simulink library "dgl_grc"  (R2024a)
settings: Solver=VariableStepAuto  StartTime=0.0  StopTime=10.0  RelTol=1e-3
undefined symbols (not defined in the file or in its folder): Diag2_bRstFault_C, Diag2_f32_UdcLowCoefAddStep_C, Diag2_f32_UdcLowCoefDepStep_C, Diag2_f32_UdcLowHysBand_C, Diag2_f32_UdcLowStartDerat_C, Diag2_f32_UdcLowStopDerat_C, Diag2_f32_UdcOverCoefAddStep_C, Diag2_f32_UdcOverCoefDepStep_C, Diag2_f32_UdcOverHysBand_C, Diag2_f32_UdcOverStartDerat_C, Diag2_f32_UdcOverStopDerat_C, Diag2_int16_HvLowErrErr_C, Diag2_int16_HvLowErrHeal_C, Diag2_int16_HvLowWarnErr_C, Diag2_int16_HvLowWarnHeal_C, Diag2_int16_HvOverErrErr_C, Diag2_int16_HvOverErrHeal_C, Diag2_int16_HvOverWarnErr_C, Diag2_int16_HvOverWarnHeal_C, DiagM_bZeroCurrMor_C, DiagM_bZeroCurrTrig_C, DiagM_Fault2LevelMor_C, DiagM_Fault2LevelTrig_C, GRC_FAKE_SAMPLE_TIME, KDGL_bBusOffEna_C, KDGL_bComInvaildVcuEna_C, KDGL_bComLostVcuEna_C, KDGL_bCurrFaultEna_C, KDGL_bEnaBenchShutDwn_C, KDGL_bEOPFaultEna_C, KDGL_bHvDcVoltFaultEna_C, KDGL_bIGNVoltFaultEna_C, KDGL_bOilTempFaultEna_C, KDGL_bPCBTempFaultEna_C, KDGL_bPosSenrFaultEna_C, KDGL_bPREREGFaultEna_C, KDGL_bRstStallPort_flg, KDGL_bSicFltFaultEna_C, KDGL_bSicTempFaultEna_C, KDGL_bTempSensrFaultEna_C, KDGL_bVCC5VFaultEna_C, KDGL_bVREF5VFaultEna_C, KDGL_bWaterTempFaultEna_C, KDGL_IGBTCoefAddStep_C, KDGL_IGBTCoefDepStep_C, KDGL_IGBTHysBand_C, KDGL_IGBTStartDerat_C, KDGL_IGBTStopDerat_C, KDGL_iMotStallProtEna_A, KDGL_MotCoefAddStep_C, KDGL_MotCoefDepStep_C, KDGL_MotHysBand_C, KDGL_MotStartDerat_C, KDGL_MotStopDerat_C, KDGL_nEOPSpdDiff_rpm, KDGL_nRotStallProtEna_rpm, KDGL_OilCoefAddStep_C, KDGL_OilCoefDepStep_C, KDGL_OilHysBand_C, KDGL_OilStartDerat_C ... (+37)
libraries: Library x28, GRC_Lib x8
(part 1 of 2)
settings Model: Creator=FVT22063  LastModifiedBy=FVT22063

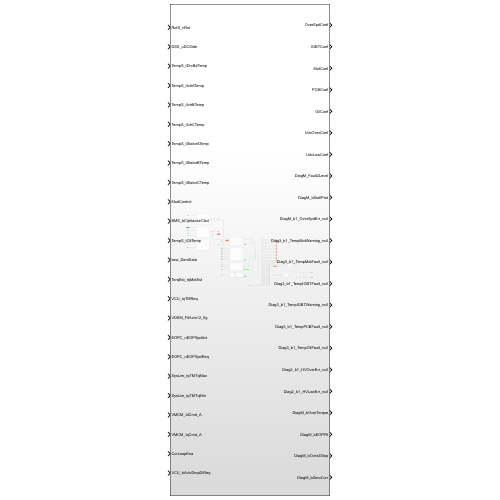
[thumbnail: Simulink's stored preview of the top-level diagram]
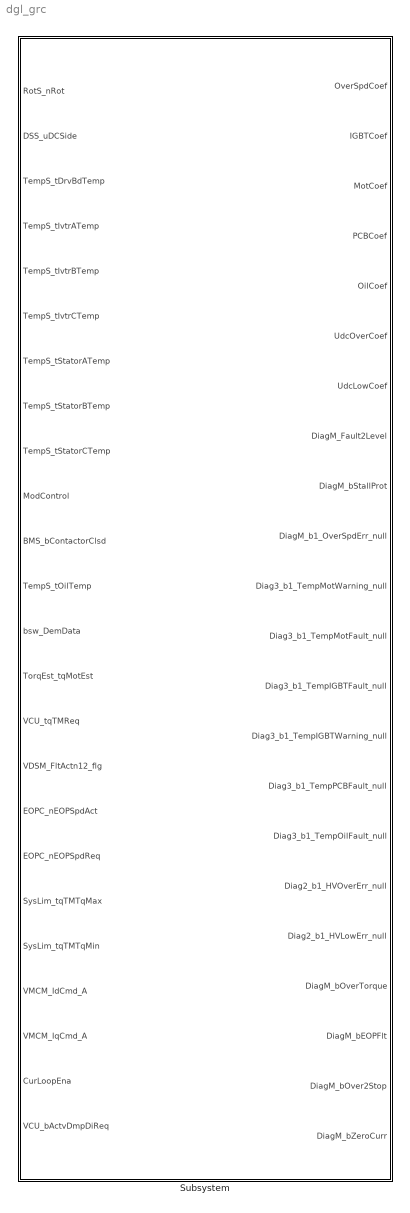
== system dgl_grc ==
  Subsystem : Subsystem

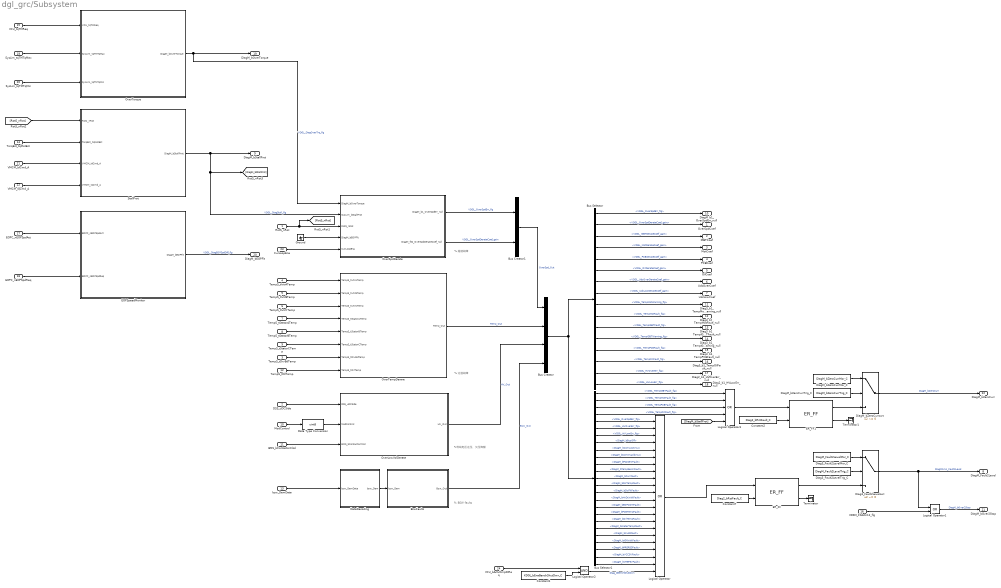
== system dgl_grc/Subsystem ==
  note: % BSW faults
  note: % 超速故障
  note: % 过温故障
  note: %母线电压过压、欠压降额
  RotS_nRot : Inport
  DSS_uDCSide : Inport  Port=2
  TempS_tDrvBdTemp : Inport  Port=3
  TempS_tIvtrATemp : Inport  Port=4
  TempS_tIvtrBTemp : Inport  Port=5
  TempS_tIvtrCTemp : Inport  Port=6
  TempS_tStatorATemp : Inport  Port=7
  TempS_tStatorBTemp : Inport  Port=8
  TempS_tStatorCTemp : Inport  Port=9
  ModControl : Inport  Port=10
  BMS_bContactorClsd : Inport  Port=11
  TempS_tOilTemp : Inport  Port=12
  bsw_DemData : Inport  Port=13  PortDimensions=150
  TorqEst_tqMotEst : Inport  Port=14
  VCU_tqTMReq : Inport  Port=15
  VDSM_FltActn12_flg : Inport  Port=16
  EOPC_nEOPSpdAct : Inport  Port=17
  EOPC_nEOPSpdReq : Inport  Port=18
  SysLim_tqTMTqMax : Inport  Port=19
  SysLim_tqTMTqMin : Inport  Port=20
  VMCM_IdCmd_A : Inport  Port=21
  VMCM_IqCmd_A : Inport  Port=22
  CurLoopEna : Inport  Port=23
  VCU_bActvDmpDiReq : Inport  Port=24
  BswFaults : Subsystem
  Bus Creator : BusCreator  Inputs=4
  Bus Creator1 : BusCreator  Inputs=2
  Bus Selector : BusSelector  OutputSignals=OverSpd_Out.VDGL_OverSpdErr_flg,OverSpd_Out.VDGL_OverSpdDerateCoef_gain,Temp_Out.IGBTTemp.VDGL_IGBTDerateCoef_gain,Temp_Out.StatorTemp.VDGL_MotDerateCoef_gain,Temp_Out.PCBTemp.VDGL_PCBDerateCoef_gain,Temp_Out.OilTemp.VDGL_OilDerateCoef_gain,HV_Out.HVOverMonitor.VDGL_UdcOverDerateCoef_gain,HV_Out.HVLowMonitor.VDGL_UdcLowDerateCoef_gain,Temp_Out.StatorTemp.VDGL_TempMotWarning_flg,Temp_Out.StatorTemp.VDGL_TempMotFault_flg,Temp_Out.IGBTTemp.VDGL_TempIGBTFault_flg,Temp_Out.IGBTTemp.VDGL_TempIGBTWarning_flg,Temp_Out.PCBTemp.VDGL_TempPCBFault_flg,Temp_Out.OilTemp.VDGL_TempOilFault_flg,HV_Out.HVOverMonitor.VDGL_HVOverErr_flg,HV_Out.HVLowMonitor.VDGL_HVLowErr_flg
  Bus Selector1 : BusSelector  OutputSignals=Temp_Out.IGBTTemp.VDGL_TempIGBTFault_flg,Temp_Out.StatorTemp.VDGL_TempMotFault_flg,Temp_Out.PCBTemp.VDGL_TempPCBFault_flg,Temp_Out.OilTemp.VDGL_TempOilFault_flg,OverSpd_Out.VDGL_OverSpdErr_flg,HV_Out.HVOverMonitor.VDGL_HVOverErr_flg,HV_Out.HVLowMonitor.VDGL_HVLowErr_flg,Bsw_Out.DiagM_bBusOff,Bsw_Out.DiagM_bComLostVcu,Bsw_Out.DiagM_bComInvaildVcu,Bsw_Out.DiagM_bPosSenrFault,Bsw_Out.DiagM_bTempSensrFault,Bsw_Out.DiagM_bCurrFault,Bsw_Out.DiagM_bSicTempFault,Bsw_Out.DiagM_bSicFltFault,Bsw_Out.DiagM_bHvDcVoltFault,Bsw_Out.DiagM_bEOPCOMFault,Bsw_Out.DiagM_bPCBTempFault,Bsw_Out.DiagM_bOilTempFault,Bsw_Out.DiagM_bWaterTempFault,Bsw_Out.DiagM_bKL30Fault,Bsw_Out.DiagM_bIGNVoltFault,Bsw_Out.DiagM_bPREREGFault,Bsw_Out.DiagM_bVCC5VFault,Bsw_Out.DiagM_bVREF5VFault
  Constant1 : Constant  Value=KDGL_bEnaBenchShutDwn_C
  Constant2 : Constant  Value=Diag2_bRstFault_C
  Constant7 : Constant  Value=Diag2_bRstFault_C
  Data Type Conversion : DataTypeConversion  OutDataTypeStr=uint8  SaturateOnIntegerOverflow=off  RndMeth=Floor
  DataDecoding : Subsystem
  Diag3_Fault2LevelMor_C : Constant  Value=DiagM_Fault2LevelMor_C
  Diag3_Fault2LevelTrig_C : Constant  Value=DiagM_Fault2LevelTrig_C
  Diag3_Fault2Levelswt : Switch  Criteria=u2 ~= 0  SaturateOnIntegerOverflow=off  InputSameDT=off
  DiagM_bZeroCurrMor_C : Constant  Value=DiagM_bZeroCurrMor_C
  DiagM_bZeroCurrTrig_C : Constant  Value=DiagM_bZeroCurrTrig_C
  DiagM_bZeroCurrswt : Switch  Criteria=u2 ~= 0  SaturateOnIntegerOverflow=off  InputSameDT=off
  EOPSpeedMonitor : Subsystem
  ER_FF : GRC_Lib/Memory/ER_FF  FalseVal=0  TrueVal=1
  ER_FF1 : GRC_Lib/Memory/ER_FF  FalseVal=0  TrueVal=1
  Ground : Ground
  Logical Operator : Logic  Operator=OR  Inputs=22  AllPortsSameDT=off  OutDataTypeStr=boolean
  Logical Operator1 : Logic  Operator=OR  AllPortsSameDT=off  OutDataTypeStr=boolean
  Logical Operator2 : Logic  AllPortsSameDT=off  OutDataTypeStr=boolean
  Logical Operator3 : Logic  Operator=OR  Inputs=5  AllPortsSameDT=off  OutDataTypeStr=boolean
  OverLowVolDerate : Subsystem
  OverSpdDerate : Subsystem
  OverTempDerare : Subsystem
  OverTorque : Subsystem
  StallProt : Subsystem
  Terminator : Terminator
  Terminator1 : Terminator
  OverSpdCoef : Outport  VectorParamsAs1DForOutWhenUnconnected=off
  IGBTCoef : Outport  Port=2  VectorParamsAs1DForOutWhenUnconnected=off
  MotCoef : Outport  Port=3  VectorParamsAs1DForOutWhenUnconnected=off
  PCBCoef : Outport  Port=4  VectorParamsAs1DForOutWhenUnconnected=off
  OilCoef : Outport  Port=5  VectorParamsAs1DForOutWhenUnconnected=off
  UdcOverCoef : Outport  Port=6  VectorParamsAs1DForOutWhenUnconnected=off
  UdcLowCoef : Outport  Port=7  VectorParamsAs1DForOutWhenUnconnected=off
  DiagM_Fault2Level : Outport  Port=8  VectorParamsAs1DForOutWhenUnconnected=off
  DiagM_bStallProt : Outport  Port=9  VectorParamsAs1DForOutWhenUnconnected=off
  DiagM_b1_OverSpdErr_null : Outport  Port=10  VectorParamsAs1DForOutWhenUnconnected=off
  Diag3_b1_TempMotWarning_null : Outport  Port=11  VectorParamsAs1DForOutWhenUnconnected=off
  Diag3_b1_TempMotFault_null : Outport  Port=12  VectorParamsAs1DForOutWhenUnconnected=off
  Diag3_b1_TempIGBTFault_null : Outport  Port=13  VectorParamsAs1DForOutWhenUnconnected=off
  Diag3_b1_TempIGBTWarning_null : Outport  Port=14  VectorParamsAs1DForOutWhenUnconnected=off
  Diag3_b1_TempPCBFault_null : Outport  Port=15  VectorParamsAs1DForOutWhenUnconnected=off
  Diag3_b1_TempOilFault_null : Outport  Port=16  VectorParamsAs1DForOutWhenUnconnected=off
  Diag2_b1_HVOverErr_null : Outport  Port=17  VectorParamsAs1DForOutWhenUnconnected=off
  Diag2_b1_HVLowErr_null : Outport  Port=18  VectorParamsAs1DForOutWhenUnconnected=off
  DiagM_bOverTorque : Outport  Port=19  VectorParamsAs1DForOutWhenUnconnected=off
  DiagM_bEOPFlt : Outport  Port=20  VectorParamsAs1DForOutWhenUnconnected=off
  DiagM_bOver2Stop : Outport  Port=21  VectorParamsAs1DForOutWhenUnconnected=off
  DiagM_bZeroCurr : Outport  Port=22  VectorParamsAs1DForOutWhenUnconnected=off
  wires:
  DiagM_bZeroCurrswt/1 -> DiagM_bZeroCurr/1  "DiagM_bZeroCurr"
  Bus Selector1/6 -> Logical Operator/2  "<VDGL_HVOverErr_flg>"
  [DiagM_bStallProt] -> Logical Operator3/5
  StallProt/1(DiagM_bStallProt) -> [DiagM_bStallProt], OverSpdDerate/2(SysLim_bStallProt), DiagM_bStallProt/1  "VDGL_DiagStall_flg"
  Bus Selector/16 -> Diag2_b1_HVLowErr_null/1  "<VDGL_HVLowErr_flg>"
  Bus Selector1/18 -> Logical Operator/14  "<DiagM_bPCBTempFault>"
  Logical Operator3/1 -> ER_FF1/1
  Bus Selector1/19 -> Logical Operator/15  "<DiagM_bOilTempFault>"
  ER_FF1/1 -> DiagM_bZeroCurrswt/3
  ER_FF1/2 -> Terminator1/1
  ER_FF/1 -> Diag3_Fault2Levelswt/3
  Bus Selector/9 -> Diag3_b1_TempMotWarning_null/1  "<VDGL_TempMotWarning_flg>"
  Diag3_Fault2LevelTrig_C/1 -> Diag3_Fault2Levelswt/2
  TempS_tStatorBTemp/1 -> OverTempDerare/5(TempS_tStatorBTemp)
  Diag3_Fault2LevelMor_C/1 -> Diag3_Fault2Levelswt/1
  VMCM_IdCmd_A/1 -> StallProt/3(VMCM_IdCmd_A)
  Ground/1 -> OverSpdDerate/4(DiagM_bEOPFlt)
  Logical Operator2/1 -> Logical Operator/22  "Diag_bBenchShutDwn"
  Bus Selector/13 -> Diag3_b1_TempPCBFault_null/1  "<VDGL_TempPCBFault_flg>"
  Constant7/1 -> ER_FF/2
  CurLoopEna/1 -> OverSpdDerate/5(CurLoopEna)
  ModControl/1 -> Data Type Conversion/1
  BswFaults/1(Bsw_Out) -> Bus Creator/4  "Bsw_Out"
  Constant1/1 -> Logical Operator2/2
  SysLim_tqTMTqMax/1 -> OverTorque/2(SysLim_tqTMTqMax)
  EOPC_nEOPSpdReq/1 -> EOPSpeedMonitor/2(EOPC_nEOPSpdReq)
  EOPSpeedMonitor/1(DiagM_bEOPFlt) -> DiagM_bEOPFlt/1  "VDGL_DiagEOPSpdDiff_flg"
  SysLim_tqTMTqMin/1 -> OverTorque/3("SysLim_tqTMTqMin ")
  EOPC_nEOPSpdAct/1 -> EOPSpeedMonitor/1(EOPC_nEOPSpdAct)
  Bus Selector/1 -> DiagM_b1_OverSpdErr_null/1  "<VDGL_OverSpdErr_flg>"
  DataDecoding/1(bsw_Dem) -> BswFaults/1(bsw_Dem)
  TorqEst_tqMotEst/1 -> StallProt/2(TorqEst_tqMotEst)
  Diag3_Fault2Levelswt/1 -> Logical Operator1/1, DiagM_Fault2Level/1  "DiagM1ms_Fault2Level"
  Bus Selector1/5 -> Logical Operator/1  "<VDGL_OverSpdErr_flg>"
  Bus Selector/12 -> Diag3_b1_TempIGBTWarning_null/1  "<VDGL_TempIGBTWarning_flg>"
  VCU_bActvDmpDiReq/1 -> Logical Operator2/1
  Logical Operator1/1 -> DiagM_bOver2Stop/1  "DiagM_bOver2Stop"
  Bus Selector1/14 -> Logical Operator/10  "<DiagM_bSicTempFault>"
  VCU_tqTMReq/1 -> OverTorque/1(VCU_tqTMReq)
  OverTorque/1(DiagM_bOverTorque) -> OverSpdDerate/1(DiagM_bOverTorque), DiagM_bOverTorque/1  "VDGL_DiagOverTrq_flg"
  DiagM_bZeroCurrMor_C/1 -> DiagM_bZeroCurrswt/1
  Bus Selector/2 -> OverSpdCoef/1  "<VDGL_OverSpdDerateCoef_gain>"
  Data Type Conversion/1 -> OverLowVolDerate/2(ModControl)
  VDSM_FltActn12_flg/1 -> Logical Operator1/2
  Bus Selector1/24 -> Logical Operator/20  "<DiagM_bVCC5VFault>"
  OverLowVolDerate/1(HV_Out) -> Bus Creator/3  "HV_Out"
  TempS_tIvtrCTemp/1 -> OverTempDerare/3(TempS_tIvtrCTemp)
  bsw_DemData/1 -> DataDecoding/1(bsw_DemData)
  ER_FF/2 -> Terminator/1
  Bus Selector1/21 -> Logical Operator/17  "<DiagM_bKL30Fault>"
  TempS_tOilTemp/1 -> OverTempDerare/8(TempS_tOilTemp)
  VMCM_IqCmd_A/1 -> StallProt/4(VMCM_IqCmd_A)
  RotS_nRot/1 -> [RotS_nRot], OverSpdDerate/3(RotS_nRot)
  Bus Selector1/12 -> Logical Operator/8  "<DiagM_bTempSensrFault>"
  Bus Selector/10 -> Diag3_b1_TempMotFault_null/1  "<VDGL_TempMotFault_flg>"
  Bus Selector1/20 -> Logical Operator/16  "<DiagM_bWaterTempFault>"
  Bus Selector1/10 -> Logical Operator/6  "<DiagM_bComInvaildVcu>"
  OverSpdDerate/2(DiagM_f32_OverSpdDerateCoef_null) -> Bus Creator1/2  "VDGL_OverSpdDerateCoef_gain"
  Bus Selector/14 -> Diag3_b1_TempOilFault_null/1  "<VDGL_TempOilFault_flg>"
  Bus Selector1/7 -> Logical Operator/3  "<VDGL_HVLowErr_flg>"
  Bus Selector1/25 -> Logical Operator/21  "<DiagM_bVREF5VFault>"
  Bus Selector1/23 -> Logical Operator/19  "<DiagM_bPREREGFault>"
  Bus Selector/15 -> Diag2_b1_HVOverErr_null/1  "<VDGL_HVOverErr_flg>"
  Bus Selector1/3 -> Logical Operator3/3  "<VDGL_TempPCBFault_flg>"
  Bus Selector/8 -> UdcLowCoef/1  "<VDGL_UdcLowDerateCoef_gain>"
  Constant2/1 -> ER_FF1/2
  OverTempDerare/1(Temp_Out) -> Bus Creator/2  "Temp_Out"
  [RotS_nRot] -> StallProt/1(Rots_nRot)
  Bus Selector1/4 -> Logical Operator3/4  "<VDGL_TempOilFault_flg>"
  Bus Selector1/17 -> Logical Operator/13  "<DiagM_bEOPCOMFault>"
  OverSpdDerate/1(DiagM_b1_OverSpdErr_null) -> Bus Creator1/1  "VDGL_OverSpdErr_flg"
  Bus Selector/5 -> PCBCoef/1  "<VDGL_PCBDerateCoef_gain>"
  TempS_tIvtrBTemp/1 -> OverTempDerare/2(TempS_tIvtrBTemp)
  BMS_bContactorClsd/1 -> OverLowVolDerate/3(BMS_bContactorClsd)
  Logical Operator/1 -> ER_FF/1
  Bus Selector1/2 -> Logical Operator3/2  "<VDGL_TempMotFault_flg>"
  Bus Selector/7 -> UdcOverCoef/1  "<VDGL_UdcOverDerateCoef_gain>"
  Bus Selector1/15 -> Logical Operator/11  "<DiagM_bSicFltFault>"
  Bus Selector1/11 -> Logical Operator/7  "<DiagM_bPosSenrFault>"
  Bus Selector/6 -> OilCoef/1  "<VDGL_OilDerateCoef_gain>"
  DSS_uDCSide/1 -> OverLowVolDerate/1(DSS_uDCSide)
  Bus Selector1/13 -> Logical Operator/9  "<DiagM_bCurrFault>"
  Bus Selector/4 -> MotCoef/1  "<VDGL_MotDerateCoef_gain>"
  Bus Selector/3 -> IGBTCoef/1  "<VDGL_IGBTDerateCoef_gain>"
  Bus Selector1/9 -> Logical Operator/5  "<DiagM_bComLostVcu>"
  Bus Selector1/16 -> Logical Operator/12  "<DiagM_bHvDcVoltFault>"
  Bus Selector1/8 -> Logical Operator/4  "<DiagM_bBusOff>"
  Bus Creator/1 -> Bus Selector1/1, Bus Selector/1
  Bus Creator1/1 -> Bus Creator/1  "OverSpd_Out"
  TempS_tStatorCTemp/1 -> OverTempDerare/6(TempS_tStatorCTemp)
  Bus Selector1/22 -> Logical Operator/18  "<DiagM_bIGNVoltFault>"
  TempS_tIvtrATemp/1 -> OverTempDerare/1(TempS_tIvtrATemp)
  DiagM_bZeroCurrTrig_C/1 -> DiagM_bZeroCurrswt/2
  TempS_tDrvBdTemp/1 -> OverTempDerare/7(TempS_tDrvBdTemp)
  Bus Selector/11 -> Diag3_b1_TempIGBTFault_null/1  "<VDGL_TempIGBTFault_flg>"
  TempS_tStatorATemp/1 -> OverTempDerare/4(TempS_tStatorATemp)
  Bus Selector1/1 -> Logical Operator3/1  "<VDGL_TempIGBTFault_flg>"

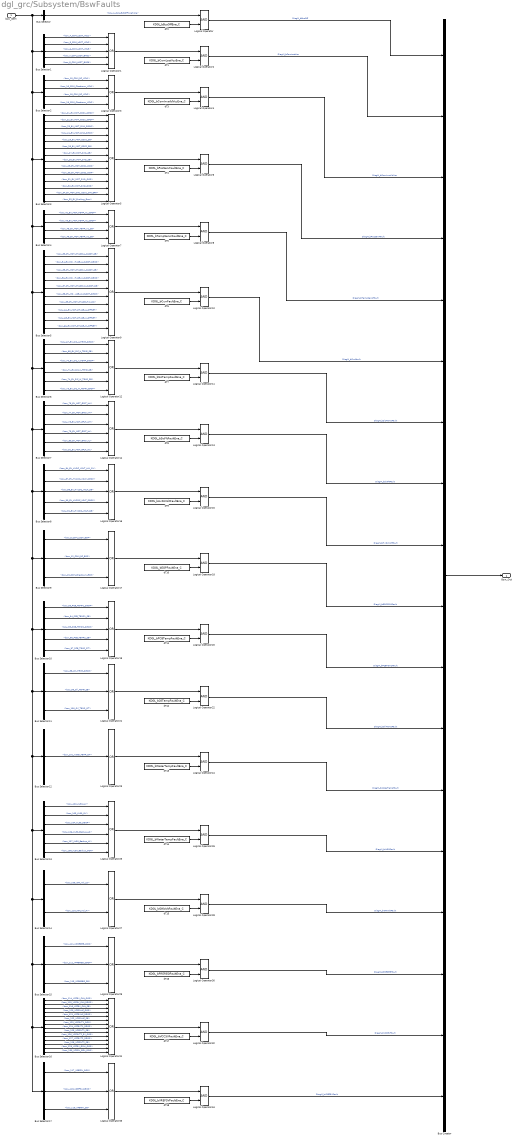
== system dgl_grc/Subsystem/BswFaults ==
  bsw_Dem : Inport
  Bus Creator : BusCreator  Inputs=18
  Bus Selector : BusSelector  OutputSignals=bsw_1_CAN_BUSOFF_Vehicle
  Bus Selector1 : BusSelector  OutputSignals=bsw_4_COM_LOST_VCU1,bsw_5_COM_LOST_VCU2,bsw_6_COM_LOST_VCU5,bsw_7_COM_LOST_BMS1,bsw_8_COM_LOST_BMS6
  Bus Selector10 : BusSelector  OutputSignals=bsw_93_PCB_TEMP1_SGOP,bsw_94_PCB_TEMP1_SB,bsw_95_PCB_TEMP2_SGOP,bsw_96_PCB_TEMP2_SB,bsw_97_PCB_TEMP_OT
  Bus Selector11 : BusSelector  OutputSignals=bsw_98_Oil_TEMP_SGOP,bsw_99_Oil_TEMP_SB,bsw_100_Oil_TEMP_OT
  Bus Selector12 : BusSelector  OutputSignals=bsw_101_water_TEMP_OT
  Bus Selector13 : BusSelector  OutputSignals=bsw_102_KL30_UV,bsw_103_KL30_OV,bsw_104_KL30_SGOP,bsw_106_KL30_Backup_LO,bsw_107_KL30_Backup_HI,bsw_108_KL30_Backup_OOR
  Bus Selector14 : BusSelector  OutputSignals=bsw_109_IGN_Vol_LO,bsw_110_IGN_Vol_HI
  Bus Selector15 : BusSelector  OutputSignals=bsw_111_VPREREG_OOR,bsw_112_VPREREG_SGOP,bsw_113_VPREREG_SB
  Bus Selector16 : BusSelector  OutputSignals=bsw_114_VCC5V_CAN_OOR,bsw_115_VCC5V_CAN_SGOP,bsw_116_VCC5V_CAN_SB,bsw_120_VCC5VUC_OOR,bsw_121_VCC5VUC_SGOP,bsw_122_VCC5VUC_SB,bsw_123_VCC5VT1_OOR,bsw_124_VCC5VT1_SGOP,bsw_125_VCC5VT1_SB,bsw_126_VCC5VT2_5V_OOR,bsw_127_VCC5VT2_SGOP,bsw_128_VCC5VT2_SB,bsw_129_VCC5V_GDH_OOR,bsw_130_VCC5V_GDL_OOR
  Bus Selector17 : BusSelector  OutputSignals=bsw_117_VREF5V_OOR,bsw_118_VREF5V_SGOP,bsw_119_VREF5V_SB
  Bus Selector2 : BusSelector  OutputSignals=bsw_15_COM_RC_VCU1,bsw_16_COM_Checksum_VCU1,bsw_18_COM_RC_VCU2,bsw_19_COM_Checksum_VCU2
  Bus Selector3 : BusSelector  OutputSignals=bsw_21_EV_MOT_COS1_SGOP,bsw_22_EV_MOT_COS2_SGOP,bsw_23_EV_MOT_SIN1_SGOP,bsw_24_EV_MOT_SIN2_SGOP,bsw_25_EV_MOT_COS1_SB,bsw_26_EV_MOT_COS2_SB,bsw_27_EV_MOT_SIN1_SB,bsw_28_EV_MOT_SIN2_SB,bsw_29_EV_MOT_COS1_OOR,bsw_30_EV_MOT_COS2_OOR,bsw_31_EV_MOT_SIN1_OOR,bsw_32_EV_MOT_SIN2_OOR,bsw_34_EV_MOT_SIN1_COS1_DIR_ERR,bsw_33_EV_Exciting_Error
  Bus Selector4 : BusSelector  OutputSignals=bsw_42_EV_MOT_TEMP_V1_SGOP,bsw_43_EV_MOT_TEMP_V2_SGOP,bsw_45_EV_MOT_TEMP_V1_SB,bsw_46_EV_MOT_TEMP_V2_SB
  Bus Selector5 : BusSelector  OutputSignals=bsw_53_EV_MOT_PHASE_U_CURRT_SB,bsw_54_EV_MOT_PHASE_U_CURRT_SGOP,bsw_55_EV_MOT_PHASE_V_CURRT_SB,bsw_56_EV_MOT_PHASE_V_CURRT_SGOP,bsw_57_EV_MOT_PHASE_W_CURRT_SB,bsw_58_EV_MOT_PHASE_W_CURRT_SGOP,bsw_59_EV_MOT_PHASE_HW_OC,bsw_64_EV_MOT_PHASE_U_OFFSET,bsw_65_EV_MOT_PHASE_V_OFFSET,bsw_66_EV_MOT_PHASE_W_OFFSET
  Bus Selector6 : BusSelector  OutputSignals=bsw_67_EV_SIC_U_TEMP_SGOP,bsw_68_EV_SIC_U_TEMP_SB,bsw_70_EV_SIC_V_TEMP_SGOP,bsw_71_EV_SIC_V_TEMP_SB,bsw_74_EV_SIC_W_TEMP_SB,bsw_73_EV_SIC_W_TEMP_SGOP
  Bus Selector7 : BusSelector  OutputSignals=bsw_76_EV_MOT_GFLT_UH,bsw_77_EV_MOT_GFLT_VH,bsw_78_EV_MOT_GFLT_WH,bsw_79_EV_MOT_GFLT_UL,bsw_80_EV_MOT_GFLT_VL,bsw_81_EV_MOT_GFLT_WL
  Bus Selector8 : BusSelector  OutputSignals=bsw_84_EV_HVDC_VOLT_HW_OV,bsw_87_EV_HV1DC_VOLT_SGOP,bsw_88_EV_HV1DC_VOLT_SB,bsw_90_EV_HV2DC_VOLT_SGOP,bsw_91_EV_HV2DC_VOLT_SB
  Bus Selector9 : BusSelector  OutputSignals=bsw_9_COM_LOST_EOP,bsw_12_COM_RC_EOP,bsw_13_COM_Checksum_EOP
  Logical Operator{,2,4,6,8,10..11,13,15,18,20,22,24,26,28,30,32,34} (18 alike) : Logic  AllPortsSameDT=off  OutDataTypeStr=boolean
  Logical Operator1 : Logic  Operator=OR  Inputs=5  AllPortsSameDT=off  OutDataTypeStr=boolean
  Logical Operator12 : Logic  Operator=OR  Inputs=6  AllPortsSameDT=off  OutDataTypeStr=boolean
  Logical Operator14 : Logic  Operator=OR  Inputs=6  AllPortsSameDT=off  OutDataTypeStr=boolean
  Logical Operator16 : Logic  Operator=OR  Inputs=5  AllPortsSameDT=off  OutDataTypeStr=boolean
  Logical Operator{17,21,29,33} (4 alike) : Logic  Operator=OR  Inputs=3  AllPortsSameDT=off  OutDataTypeStr=boolean
  Logical Operator19 : Logic  Operator=OR  Inputs=5  AllPortsSameDT=off  OutDataTypeStr=boolean
  Logical Operator23 : Logic  Operator=OR  Inputs=1  AllPortsSameDT=off  OutDataTypeStr=boolean
  Logical Operator25 : Logic  Operator=OR  Inputs=6  AllPortsSameDT=off  OutDataTypeStr=boolean
  Logical Operator27 : Logic  Operator=OR  AllPortsSameDT=off  OutDataTypeStr=boolean
  Logical Operator3 : Logic  Operator=OR  Inputs=4  AllPortsSameDT=off  OutDataTypeStr=boolean
  Logical Operator31 : Logic  Operator=OR  Inputs=14  AllPortsSameDT=off  OutDataTypeStr=boolean
  Logical Operator5 : Logic  Operator=OR  Inputs=14  AllPortsSameDT=off  OutDataTypeStr=boolean
  Logical Operator7 : Logic  Operator=OR  Inputs=4  AllPortsSameDT=off  OutDataTypeStr=boolean
  Logical Operator9 : Logic  Operator=OR  Inputs=10  AllPortsSameDT=off  OutDataTypeStr=boolean
  dT1 : Constant  Value=KDGL_bComLostVcuEna_C  OutDataTypeStr=single
  dT10 : Constant  Value=KDGL_bEOPFaultEna_C  OutDataTypeStr=single
  dT11 : Constant  Value=KDGL_bPCBTempFaultEna_C  OutDataTypeStr=single
  dT12 : Constant  Value=KDGL_bOilTempFaultEna_C  OutDataTypeStr=single
  dT13 : Constant  Value=KDGL_bWaterTempFaultEna_C  OutDataTypeStr=single
  dT14 : Constant  Value=KDGL_bWaterTempFaultEna_C  OutDataTypeStr=single
  dT15 : Constant  Value=KDGL_bIGNVoltFaultEna_C  OutDataTypeStr=single
  dT16 : Constant  Value=KDGL_bPREREGFaultEna_C  OutDataTypeStr=single
  dT17 : Constant  Value=KDGL_bVCC5VFaultEna_C  OutDataTypeStr=single
  dT18 : Constant  Value=KDGL_bVREF5VFaultEna_C  OutDataTypeStr=single
  dT2 : Constant  Value=KDGL_bBusOffEna_C  OutDataTypeStr=single
  dT3 : Constant  Value=KDGL_bComInvaildVcuEna_C  OutDataTypeStr=single
  dT4 : Constant  Value=KDGL_bPosSenrFaultEna_C  OutDataTypeStr=single
  dT5 : Constant  Value=KDGL_bTempSensrFaultEna_C  OutDataTypeStr=single
  dT6 : Constant  Value=KDGL_bCurrFaultEna_C  OutDataTypeStr=single
  dT7 : Constant  Value=KDGL_bSicTempFaultEna_C  OutDataTypeStr=single
  dT8 : Constant  Value=KDGL_bSicFltFaultEna_C  OutDataTypeStr=single
  dT9 : Constant  Value=KDGL_bHvDcVoltFaultEna_C  OutDataTypeStr=single
  Bsw_Out : Outport  VectorParamsAs1DForOutWhenUnconnected=off
  wires:
  Bus Creator/1 -> Bsw_Out/1
  Bus Selector/1 -> Logical Operator/1  "<bsw_1_CAN_BUSOFF_Vehicle>"
  Logical Operator/1 -> Bus Creator/1  "DiagM_bBusOff"
  dT2/1 -> Logical Operator/2
  Bus Selector1/1 -> Logical Operator1/1  "<bsw_4_COM_LOST_VCU1>"
  Bus Selector1/2 -> Logical Operator1/2  "<bsw_5_COM_LOST_VCU2>"
  Bus Selector1/3 -> Logical Operator1/3  "<bsw_6_COM_LOST_VCU5>"
  Bus Selector1/4 -> Logical Operator1/4  "<bsw_7_COM_LOST_BMS1>"
  Bus Selector1/5 -> Logical Operator1/5  "<bsw_8_COM_LOST_BMS6>"
  dT1/1 -> Logical Operator2/2
  Logical Operator1/1 -> Logical Operator2/1
  Logical Operator2/1 -> Bus Creator/2  "DiagM_bComLostVcu"
  Bus Selector2/3 -> Logical Operator3/3  "<bsw_18_COM_RC_VCU2>"
  Bus Selector2/2 -> Logical Operator3/2  "<bsw_16_COM_Checksum_VCU1>"
  Bus Selector2/4 -> Logical Operator3/4  "<bsw_19_COM_Checksum_VCU2>"
  Bus Selector2/1 -> Logical Operator3/1  "<bsw_15_COM_RC_VCU1>"
  dT3/1 -> Logical Operator4/2
  Logical Operator3/1 -> Logical Operator4/1
  Logical Operator4/1 -> Bus Creator/3  "DiagM_bComInvaildVcu"
  Bus Selector3/1 -> Logical Operator5/1  "<bsw_21_EV_MOT_COS1_SGOP>"
  Bus Selector3/2 -> Logical Operator5/2  "<bsw_22_EV_MOT_COS2_SGOP>"
  Bus Selector3/3 -> Logical Operator5/3  "<bsw_23_EV_MOT_SIN1_SGOP>"
  Bus Selector3/4 -> Logical Operator5/4  "<bsw_24_EV_MOT_SIN2_SGOP>"
  Bus Selector3/5 -> Logical Operator5/5  "<bsw_25_EV_MOT_COS1_SB>"
  Bus Selector3/6 -> Logical Operator5/6  "<bsw_26_EV_MOT_COS2_SB>"
  Bus Selector3/7 -> Logical Operator5/7  "<bsw_27_EV_MOT_SIN1_SB>"
  Bus Selector3/8 -> Logical Operator5/8  "<bsw_28_EV_MOT_SIN2_SB>"
  Bus Selector3/9 -> Logical Operator5/9  "<bsw_29_EV_MOT_COS1_OOR>"
  Bus Selector3/10 -> Logical Operator5/10  "<bsw_30_EV_MOT_COS2_OOR>"
  Bus Selector3/11 -> Logical Operator5/11  "<bsw_31_EV_MOT_SIN1_OOR>"
  Bus Selector3/12 -> Logical Operator5/12  "<bsw_32_EV_MOT_SIN2_OOR>"
  dT4/1 -> Logical Operator6/2
  Logical Operator5/1 -> Logical Operator6/1
  Logical Operator6/1 -> Bus Creator/4  "DiagM_bPosSenrFault"
  Bus Selector3/13 -> Logical Operator5/13  "<bsw_34_EV_MOT_SIN1_COS1_DIR_ERR>"
  Bus Selector3/14 -> Logical Operator5/14  "<bsw_33_EV_Exciting_Error>"
  Logical Operator7/1 -> Logical Operator8/1
  dT5/1 -> Logical Operator8/2
  Bus Selector4/1 -> Logical Operator7/1  "<bsw_42_EV_MOT_TEMP_V1_SGOP>"
  Bus Selector4/4 -> Logical Operator7/4  "<bsw_46_EV_MOT_TEMP_V2_SB>"
  Bus Selector4/2 -> Logical Operator7/2  "<bsw_43_EV_MOT_TEMP_V2_SGOP>"
  Bus Selector4/3 -> Logical Operator7/3  "<bsw_45_EV_MOT_TEMP_V1_SB>"
  bsw_Dem/1 -> Bus Selector17/1, Bus Selector16/1, Bus Selector15/1, Bus Selector14/1, Bus Selector13/1, Bus Selector12/1, Bus Selector11/1, Bus Selector10/1, Bus Selector9/1, Bus Selector8/1, Bus Selector7/1, Bus Selector6/1, Bus Selector5/1, Bus Selector4/1, Bus Selector3/1, Bus Selector2/1, Bus Selector1/1, Bus Selector/1
  Logical Operator8/1 -> Bus Creator/5  "DiagM_bTempSensrFault"
  Bus Selector5/1 -> Logical Operator9/1  "<bsw_53_EV_MOT_PHASE_U_CURRT_SB>"
  Bus Selector5/2 -> Logical Operator9/2  "<bsw_54_EV_MOT_PHASE_U_CURRT_SGOP>"
  Bus Selector5/3 -> Logical Operator9/3  "<bsw_55_EV_MOT_PHASE_V_CURRT_SB>"
  Bus Selector5/4 -> Logical Operator9/4  "<bsw_56_EV_MOT_PHASE_V_CURRT_SGOP>"
  Bus Selector5/5 -> Logical Operator9/5  "<bsw_57_EV_MOT_PHASE_W_CURRT_SB>"
  Bus Selector5/6 -> Logical Operator9/6  "<bsw_58_EV_MOT_PHASE_W_CURRT_SGOP>"
  Bus Selector5/7 -> Logical Operator9/7  "<bsw_59_EV_MOT_PHASE_HW_OC>"
  Bus Selector5/8 -> Logical Operator9/8  "<bsw_64_EV_MOT_PHASE_U_OFFSET>"
  Bus Selector5/9 -> Logical Operator9/9  "<bsw_65_EV_MOT_PHASE_V_OFFSET>"
  Bus Selector5/10 -> Logical Operator9/10  "<bsw_66_EV_MOT_PHASE_W_OFFSET>"
  dT6/1 -> Logical Operator10/2
  Logical Operator9/1 -> Logical Operator10/1
  Logical Operator10/1 -> Bus Creator/6  "DiagM_bCurrFault"
  Logical Operator12/1 -> Logical Operator11/1
  dT7/1 -> Logical Operator11/2
  Bus Selector6/6 -> Logical Operator12/6  "<bsw_73_EV_SIC_W_TEMP_SGOP>"
  Bus Selector6/5 -> Logical Operator12/5  "<bsw_74_EV_SIC_W_TEMP_SB>"
  Bus Selector6/4 -> Logical Operator12/4  "<bsw_71_EV_SIC_V_TEMP_SB>"
  Bus Selector6/3 -> Logical Operator12/3  "<bsw_70_EV_SIC_V_TEMP_SGOP>"
  Bus Selector6/2 -> Logical Operator12/2  "<bsw_68_EV_SIC_U_TEMP_SB>"
  Bus Selector6/1 -> Logical Operator12/1  "<bsw_67_EV_SIC_U_TEMP_SGOP>"
  Logical Operator11/1 -> Bus Creator/7  "DiagM_bSicTempFault"
  Bus Selector7/1 -> Logical Operator14/1  "<bsw_76_EV_MOT_GFLT_UH>"
  Bus Selector7/2 -> Logical Operator14/2  "<bsw_77_EV_MOT_GFLT_VH>"
  Bus Selector7/3 -> Logical Operator14/3  "<bsw_78_EV_MOT_GFLT_WH>"
  Bus Selector7/4 -> Logical Operator14/4  "<bsw_79_EV_MOT_GFLT_UL>"
  Bus Selector7/5 -> Logical Operator14/5  "<bsw_80_EV_MOT_GFLT_VL>"
  Bus Selector7/6 -> Logical Operator14/6  "<bsw_81_EV_MOT_GFLT_WL>"
  dT8/1 -> Logical Operator13/2
  Logical Operator14/1 -> Logical Operator13/1
  Logical Operator13/1 -> Bus Creator/8  "DiagM_bSicFltFault"
  Logical Operator16/1 -> Logical Operator15/1
  dT9/1 -> Logical Operator15/2
  Bus Selector8/5 -> Logical Operator16/5  "<bsw_91_EV_HV2DC_VOLT_SB>"
  Bus Selector8/4 -> Logical Operator16/4  "<bsw_90_EV_HV2DC_VOLT_SGOP>"
  Bus Selector8/3 -> Logical Operator16/3  "<bsw_88_EV_HV1DC_VOLT_SB>"
  Bus Selector8/2 -> Logical Operator16/2  "<bsw_87_EV_HV1DC_VOLT_SGOP>"
  Bus Selector8/1 -> Logical Operator16/1  "<bsw_84_EV_HVDC_VOLT_HW_OV>"
  Logical Operator15/1 -> Bus Creator/9  "DiagM_bHvDcVoltFault"
  Bus Selector9/1 -> Logical Operator17/1  "<bsw_9_COM_LOST_EOP>"
  Bus Selector9/2 -> Logical Operator17/2  "<bsw_12_COM_RC_EOP>"
  Bus Selector9/3 -> Logical Operator17/3  "<bsw_13_COM_Checksum_EOP>"
  Logical Operator17/1 -> Logical Operator18/1
  dT10/1 -> Logical Operator18/2
  Logical Operator18/1 -> Bus Creator/10  "DiagM_bEOPCOMFault"
  Bus Selector10/1 -> Logical Operator19/1  "<bsw_93_PCB_TEMP1_SGOP>"
  Bus Selector10/2 -> Logical Operator19/2  "<bsw_94_PCB_TEMP1_SB>"
  Bus Selector10/3 -> Logical Operator19/3  "<bsw_95_PCB_TEMP2_SGOP>"
  Bus Selector10/4 -> Logical Operator19/4  "<bsw_96_PCB_TEMP2_SB>"
  Bus Selector10/5 -> Logical Operator19/5  "<bsw_97_PCB_TEMP_OT>"
  Logical Operator19/1 -> Logical Operator20/1
  dT11/1 -> Logical Operator20/2
  Logical Operator20/1 -> Bus Creator/11  "DiagM_bPCBTempFault"
  Bus Selector11/1 -> Logical Operator21/1  "<bsw_98_Oil_TEMP_SGOP>"
  Bus Selector11/2 -> Logical Operator21/2  "<bsw_99_Oil_TEMP_SB>"
  Bus Selector11/3 -> Logical Operator21/3  "<bsw_100_Oil_TEMP_OT>"
  Logical Operator21/1 -> Logical Operator22/1
  dT12/1 -> Logical Operator22/2
  Logical Operator22/1 -> Bus Creator/12  "DiagM_bOilTempFault"
  Bus Selector12/1 -> Logical Operator23/1  "<bsw_101_water_TEMP_OT>"
  Logical Operator23/1 -> Logical Operator24/1
  dT13/1 -> Logical Operator24/2
  Logical Operator24/1 -> Bus Creator/13  "DiagM_bWaterTempFault"
  Bus Selector13/1 -> Logical Operator25/1  "<bsw_102_KL30_UV>"
  Bus Selector13/2 -> Logical Operator25/2  "<bsw_103_KL30_OV>"
  Bus Selector13/3 -> Logical Operator25/3  "<bsw_104_KL30_SGOP>"
  Bus Selector13/4 -> Logical Operator25/4  "<bsw_106_KL30_Backup_LO>"
  Bus Selector13/5 -> Logical Operator25/5  "<bsw_107_KL30_Backup_HI>"
  Bus Selector13/6 -> Logical Operator25/6  "<bsw_108_KL30_Backup_OOR>"
  Logical Operator25/1 -> Logical Operator26/1
  dT14/1 -> Logical Operator26/2
  Logical Operator26/1 -> Bus Creator/14  "DiagM_bKL30Fault"
  Bus Selector14/1 -> Logical Operator27/1  "<bsw_109_IGN_Vol_LO>"
  Bus Selector14/2 -> Logical Operator27/2  "<bsw_110_IGN_Vol_HI>"
  Logical Operator27/1 -> Logical Operator28/1
  dT15/1 -> Logical Operator28/2
  Logical Operator28/1 -> Bus Creator/15  "DiagM_bIGNVoltFault"
  Bus Selector15/1 -> Logical Operator29/1  "<bsw_111_VPREREG_OOR>"
  Bus Selector15/2 -> Logical Operator29/2  "<bsw_112_VPREREG_SGOP>"
  Bus Selector15/3 -> Logical Operator29/3  "<bsw_113_VPREREG_SB>"
  Logical Operator29/1 -> Logical Operator30/1
  dT16/1 -> Logical Operator30/2
  Logical Operator30/1 -> Bus Creator/16  "DiagM_bPREREGFault"
  Bus Selector16/1 -> Logical Operator31/1  "<bsw_114_VCC5V_CAN_OOR>"
  Bus Selector16/2 -> Logical Operator31/2  "<bsw_115_VCC5V_CAN_SGOP>"
  Bus Selector16/3 -> Logical Operator31/3  "<bsw_116_VCC5V_CAN_SB>"
  Bus Selector16/4 -> Logical Operator31/4  "<bsw_120_VCC5VUC_OOR>"
  Bus Selector16/5 -> Logical Operator31/5  "<bsw_121_VCC5VUC_SGOP>"
  Bus Selector16/6 -> Logical Operator31/6  "<bsw_122_VCC5VUC_SB>"
  Bus Selector16/7 -> Logical Operator31/7  "<bsw_123_VCC5VT1_OOR>"
  Bus Selector16/8 -> Logical Operator31/8  "<bsw_124_VCC5VT1_SGOP>"
  Bus Selector16/9 -> Logical Operator31/9  "<bsw_125_VCC5VT1_SB>"
  Bus Selector16/10 -> Logical Operator31/10  "<bsw_126_VCC5VT2_5V_OOR>"
  Bus Selector16/11 -> Logical Operator31/11  "<bsw_127_VCC5VT2_SGOP>"
  Bus Selector16/12 -> Logical Operator31/12  "<bsw_128_VCC5VT2_SB>"
  Bus Selector16/13 -> Logical Operator31/13  "<bsw_129_VCC5V_GDH_OOR>"
  Bus Selector16/14 -> Logical Operator31/14  "<bsw_130_VCC5V_GDL_OOR>"
  Logical Operator31/1 -> Logical Operator32/1
  dT17/1 -> Logical Operator32/2
  Logical Operator32/1 -> Bus Creator/17  "DiagM_bVCC5VFault"
  Bus Selector17/1 -> Logical Operator33/1  "<bsw_117_VREF5V_OOR>"
  Bus Selector17/2 -> Logical Operator33/2  "<bsw_118_VREF5V_SGOP>"
  Bus Selector17/3 -> Logical Operator33/3  "<bsw_119_VREF5V_SB>"
  Logical Operator33/1 -> Logical Operator34/1
  dT18/1 -> Logical Operator34/2
  Logical Operator34/1 -> Bus Creator/18  "DiagM_bVREF5VFault"

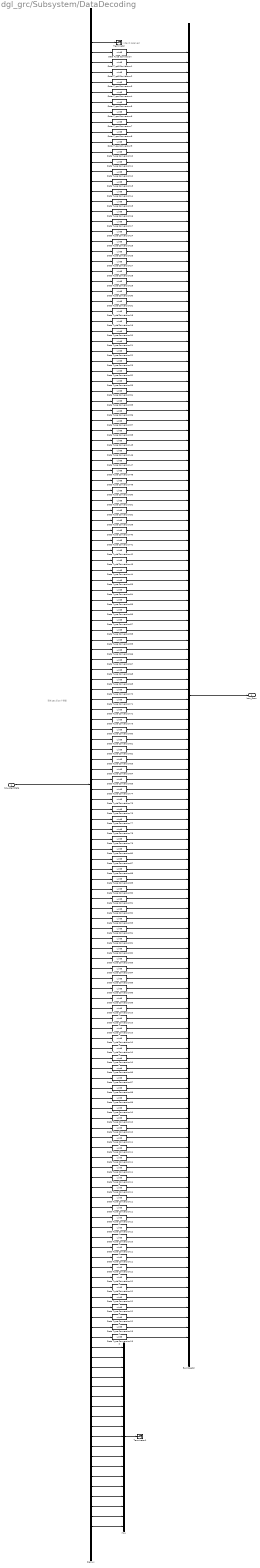
== system dgl_grc/Subsystem/DataDecoding ==
  note: index0 reserved
  note: 取前131
      | 后19个预留
  bsw_DemData : Inport  OutDataTypeStr=uint8  PortDimensions=150
  Bus Creator : BusCreator  Inputs=130
  Data Type Conversion{,1..121,124..129,131..132} (130 alike) : DataTypeConversion  OutDataTypeStr=uint8  SaturateOnIntegerOverflow=off  RndMeth=Floor
  Demux : Demux  Outputs=150
  Mux : Mux  Inputs=19
  Terminator : Terminator
  Terminator1 : Terminator
  bsw_Dem : Outport  VectorParamsAs1DForOutWhenUnconnected=off
  wires:
  bsw_DemData/1 -> Demux/1  "bsw_DemDataLo"
  Demux/1 -> Terminator/1
  Demux/2 -> Data Type Conversion/1
  Demux/3 -> Data Type Conversion1/1
  Demux/4 -> Data Type Conversion2/1
  Demux/5 -> Data Type Conversion3/1
  Demux/6 -> Data Type Conversion4/1
  Demux/7 -> Data Type Conversion5/1
  Demux/8 -> Data Type Conversion6/1
  Demux/9 -> Data Type Conversion7/1
  Demux/10 -> Data Type Conversion8/1
  Demux/11 -> Data Type Conversion9/1
  Demux/12 -> Data Type Conversion10/1
  Demux/13 -> Data Type Conversion11/1
  Demux/14 -> Data Type Conversion12/1
  Demux/15 -> Data Type Conversion13/1
  Demux/16 -> Data Type Conversion14/1
  Demux/17 -> Data Type Conversion15/1
  Demux/18 -> Data Type Conversion16/1
  Demux/19 -> Data Type Conversion17/1
  Demux/20 -> Data Type Conversion24/1
  Demux/21 -> Data Type Conversion25/1
  Demux/22 -> Data Type Conversion26/1
  Demux/23 -> Data Type Conversion27/1
  Demux/24 -> Data Type Conversion28/1
  Demux/25 -> Data Type Conversion29/1
  Demux/26 -> Data Type Conversion30/1
  Demux/27 -> Data Type Conversion31/1
  Demux/28 -> Data Type Conversion18/1
  Demux/29 -> Data Type Conversion19/1
  Demux/30 -> Data Type Conversion20/1
  Demux/31 -> Data Type Conversion21/1
  Demux/32 -> Data Type Conversion22/1
  Demux/33 -> Data Type Conversion23/1
  Demux/34 -> Data Type Conversion32/1
  Demux/35 -> Data Type Conversion33/1
  Demux/36 -> Data Type Conversion34/1
  Demux/37 -> Data Type Conversion35/1
  Demux/38 -> Data Type Conversion36/1
  Demux/39 -> Data Type Conversion37/1
  Demux/40 -> Data Type Conversion38/1
  Demux/41 -> Data Type Conversion45/1
  Demux/42 -> Data Type Conversion46/1
  Demux/43 -> Data Type Conversion47/1
  Demux/44 -> Data Type Conversion48/1
  Demux/45 -> Data Type Conversion49/1
  Demux/46 -> Data Type Conversion50/1
  Demux/47 -> Data Type Conversion51/1
  Demux/48 -> Data Type Conversion52/1
  Demux/49 -> Data Type Conversion39/1
  Demux/50 -> Data Type Conversion40/1
  Demux/51 -> Data Type Conversion41/1
  Demux/52 -> Data Type Conversion42/1
  Demux/53 -> Data Type Conversion43/1
  Demux/54 -> Data Type Conversion44/1
  Demux/55 -> Data Type Conversion53/1
  Demux/56 -> Data Type Conversion54/1
  Demux/57 -> Data Type Conversion55/1
  Demux/58 -> Data Type Conversion56/1
  Demux/59 -> Data Type Conversion57/1
  Demux/60 -> Data Type Conversion58/1
  Demux/61 -> Data Type Conversion59/1
  Demux/62 -> Data Type Conversion66/1
  Demux/63 -> Data Type Conversion67/1
  Demux/64 -> Data Type Conversion68/1
  Demux/65 -> Data Type Conversion69/1
  Demux/66 -> Data Type Conversion70/1
  Demux/67 -> Data Type Conversion71/1
  Demux/68 -> Data Type Conversion72/1
  Demux/69 -> Data Type Conversion73/1
  Demux/70 -> Data Type Conversion60/1
  Demux/71 -> Data Type Conversion61/1
  Demux/72 -> Data Type Conversion62/1
  Demux/73 -> Data Type Conversion63/1
  Demux/74 -> Data Type Conversion64/1
  Demux/75 -> Data Type Conversion65/1
  Demux/76 -> Data Type Conversion74/1
  Demux/77 -> Data Type Conversion75/1
  Demux/78 -> Data Type Conversion76/1
  Demux/79 -> Data Type Conversion77/1
  Demux/80 -> Data Type Conversion78/1
  Demux/81 -> Data Type Conversion79/1
  Demux/82 -> Data Type Conversion80/1
  Demux/83 -> Data Type Conversion87/1
  Demux/84 -> Data Type Conversion88/1
  Demux/85 -> Data Type Conversion89/1
  Demux/86 -> Data Type Conversion90/1
  Demux/87 -> Data Type Conversion91/1
  Demux/88 -> Data Type Conversion92/1
  Demux/89 -> Data Type Conversion93/1
  Demux/90 -> Data Type Conversion94/1
  Demux/91 -> Data Type Conversion81/1
  Demux/92 -> Data Type Conversion82/1
  Demux/93 -> Data Type Conversion83/1
  Demux/94 -> Data Type Conversion84/1
  Demux/95 -> Data Type Conversion85/1
  Demux/96 -> Data Type Conversion86/1
  Demux/97 -> Data Type Conversion95/1
  Demux/98 -> Data Type Conversion102/1
  Demux/99 -> Data Type Conversion103/1
  Demux/100 -> Data Type Conversion104/1
  Demux/101 -> Data Type Conversion105/1
  Demux/102 -> Data Type Conversion106/1
  Demux/103 -> Data Type Conversion107/1
  Demux/104 -> Data Type Conversion96/1
  Demux/105 -> Data Type Conversion97/1
  Demux/106 -> Data Type Conversion98/1
  Demux/107 -> Data Type Conversion99/1
  Demux/108 -> Data Type Conversion100/1
  Demux/109 -> Data Type Conversion101/1
  Demux/110 -> Data Type Conversion108/1
  Demux/111 -> Data Type Conversion111/1
  Demux/112 -> Data Type Conversion112/1
  Demux/113 -> Data Type Conversion113/1
  Demux/114 -> Data Type Conversion114/1
  Demux/115 -> Data Type Conversion115/1
  Demux/116 -> Data Type Conversion116/1
  Demux/117 -> Data Type Conversion118/1
  Demux/118 -> Data Type Conversion119/1
  Demux/119 -> Data Type Conversion120/1
  Demux/120 -> Data Type Conversion121/1
  Demux/121 -> Data Type Conversion109/1
  Demux/122 -> Data Type Conversion110/1
  Demux/123 -> Data Type Conversion117/1
  Demux/124 -> Data Type Conversion124/1
  Demux/125 -> Data Type Conversion125/1
  Demux/126 -> Data Type Conversion126/1
  Demux/127 -> Data Type Conversion127/1
  Demux/128 -> Data Type Conversion128/1
  Demux/129 -> Data Type Conversion129/1
  Demux/130 -> Data Type Conversion131/1
  Demux/131 -> Data Type Conversion132/1
  Bus Creator/1 -> bsw_Dem/1
  Data Type Conversion/1 -> Bus Creator/1  "bsw_1_CAN_BUSOFF_Vehicle"
  Data Type Conversion1/1 -> Bus Creator/2  "bsw_2_CAN_COM_LOST_xxx"
  Data Type Conversion2/1 -> Bus Creator/3  "bsw_3_CAN_COM_xxx"
  Data Type Conversion3/1 -> Bus Creator/4  "bsw_4_COM_LOST_VCU1"
  Data Type Conversion7/1 -> Bus Creator/8  "bsw_8_COM_LOST_BMS6"
  Data Type Conversion5/1 -> Bus Creator/6  "bsw_6_COM_LOST_VCU5"
  Data Type Conversion6/1 -> Bus Creator/7  "bsw_7_COM_LOST_BMS1"
  Data Type Conversion4/1 -> Bus Creator/5  "bsw_5_COM_LOST_VCU2"
  Data Type Conversion8/1 -> Bus Creator/9  "bsw_9_COM_LOST_EOP"
  Data Type Conversion9/1 -> Bus Creator/10  "bsw_10_COM_LOST_THCM1"
  Data Type Conversion11/1 -> Bus Creator/12  "bsw_12_COM_RC_EOP"
  Data Type Conversion10/1 -> Bus Creator/11  "bsw_11_COM_LOST_GW3"
  Data Type Conversion14/1 -> Bus Creator/15  "bsw_15_COM_RC_VCU1"
  Data Type Conversion12/1 -> Bus Creator/13  "bsw_13_COM_Checksum_EOP"
  Data Type Conversion13/1 -> Bus Creator/14  "bsw_14_COM_E2E_EOP"
  Data Type Conversion15/1 -> Bus Creator/16  "bsw_16_COM_Checksum_VCU1"
  Data Type Conversion16/1 -> Bus Creator/17  "bsw_17_COM_E2E_VCU1"
  Data Type Conversion20/1 -> Bus Creator/29  "bsw_29_EV_MOT_COS1_OOR"
  Data Type Conversion18/1 -> Bus Creator/27  "bsw_27_EV_MOT_SIN1_SB"
  Data Type Conversion21/1 -> Bus Creator/30  "bsw_30_EV_MOT_COS2_OOR"
  Data Type Conversion17/1 -> Bus Creator/18  "bsw_18_COM_RC_VCU2"
  Data Type Conversion22/1 -> Bus Creator/31  "bsw_31_EV_MOT_SIN1_OOR"
  Data Type Conversion19/1 -> Bus Creator/28  "bsw_28_EV_MOT_SIN2_SB"
  Data Type Conversion25/1 -> Bus Creator/20  "bsw_20_COM_E2E_VCU2"
  Data Type Conversion24/1 -> Bus Creator/19  "bsw_19_COM_Checksum_VCU2"
  Data Type Conversion23/1 -> Bus Creator/32  "bsw_32_EV_MOT_SIN2_OOR"
  Data Type Conversion27/1 -> Bus Creator/22  "bsw_22_EV_MOT_COS2_SGOP"
  Data Type Conversion26/1 -> Bus Creator/21  "bsw_21_EV_MOT_COS1_SGOP"
  Data Type Conversion28/1 -> Bus Creator/23  "bsw_23_EV_MOT_SIN1_SGOP"
  Data Type Conversion30/1 -> Bus Creator/25  "bsw_25_EV_MOT_COS1_SB"
  Data Type Conversion29/1 -> Bus Creator/24  "bsw_24_EV_MOT_SIN2_SGOP"
  Data Type Conversion31/1 -> Bus Creator/26  "bsw_26_EV_MOT_COS2_SB"
  Data Type Conversion32/1 -> Bus Creator/33  "bsw_33_EV_Exciting_Error"
  Data Type Conversion33/1 -> Bus Creator/34  "bsw_34_EV_MOT_SIN1_COS1_DIR_ERR"
  Data Type Conversion34/1 -> Bus Creator/35  "bsw_35"
  Data Type Conversion35/1 -> Bus Creator/36  "bsw_36"
  Data Type Conversion36/1 -> Bus Creator/37  "bsw_37"
  Data Type Conversion39/1 -> Bus Creator/48  "bsw_48_EV_MOT_U_OOR"
  Data Type Conversion38/1 -> Bus Creator/39  "bsw_39"
  Data Type Conversion40/1 -> Bus Creator/49  "bsw_49_EV_MOT_V_OOR"
  Data Type Conversion37/1 -> Bus Creator/38  "bsw_38"
  Data Type Conversion41/1 -> Bus Creator/50  "bsw_50_EV_MOT_W_OOR"
  Data Type Conversion45/1 -> Bus Creator/40  "bsw_40_EV_MOT_OVER_SPEED"
  Data Type Conversion43/1 -> Bus Creator/52  "bsw_52_EV_MOT_CRIT_OT"
  Data Type Conversion44/1 -> Bus Creator/53  "bsw_53_EV_MOT_PHASE_U_CURRT_SB"
  Data Type Conversion42/1 -> Bus Creator/51  "bsw_51_EV_MOT_OT"
  Data Type Conversion47/1 -> Bus Creator/42  "bsw_42_EV_MOT_TEMP_V1_SGOP"
  Data Type Conversion50/1 -> Bus Creator/45  "bsw_45_EV_MOT_TEMP_V1_SB"
  Data Type Conversion49/1 -> Bus Creator/44  "bsw_44_EV_MOT_TEMP_W_SGOP"
  Data Type Conversion46/1 -> Bus Creator/41  "bsw_41_EV_MOT_STUCK"
  Data Type Conversion48/1 -> Bus Creator/43  "bsw_43_EV_MOT_TEMP_V2_SGOP"
  Data Type Conversion52/1 -> Bus Creator/47  "bsw_47_EV_MOT_TEMP_W_SB"
  Data Type Conversion51/1 -> Bus Creator/46  "bsw_46_EV_MOT_TEMP_V2_SB"
  Data Type Conversion53/1 -> Bus Creator/54  "bsw_54_EV_MOT_PHASE_U_CURRT_SGOP"
  Data Type Conversion56/1 -> Bus Creator/57  "bsw_57_EV_MOT_PHASE_W_CURRT_SB"
  Data Type Conversion55/1 -> Bus Creator/56  "bsw_56_EV_MOT_PHASE_V_CURRT_SGOP"
  Data Type Conversion54/1 -> Bus Creator/55  "bsw_55_EV_MOT_PHASE_V_CURRT_SB"
  Data Type Conversion58/1 -> Bus Creator/59  "bsw_59_EV_MOT_PHASE_HW_OC"
  Data Type Conversion61/1 -> Bus Creator/70  "bsw_70_EV_SIC_V_TEMP_SGOP"
  Data Type Conversion60/1 -> Bus Creator/69  "bsw_69_EV_SIC_U_TEMP_OOR"
  Data Type Conversion59/1 -> Bus Creator/60  "bsw_60_EV_MOT_PHASE_U_SW_OC"
  Data Type Conversion57/1 -> Bus Creator/58  "bsw_58_EV_MOT_PHASE_W_CURRT_SGOP"
  Data Type Conversion63/1 -> Bus Creator/72  "bsw_72_EV_SIC_V_TEMP_OOR"
  Data Type Conversion62/1 -> Bus Creator/71  "bsw_71_EV_SIC_V_TEMP_SB"
  Data Type Conversion64/1 -> Bus Creator/73  "bsw_73_EV_SIC_W_TEMP_SGOP"
  Data Type Conversion66/1 -> Bus Creator/61  "bsw_61_EV_MOT_PHASE_V_SW_OC"
  Data Type Conversion65/1 -> Bus Creator/74  "bsw_74_EV_SIC_W_TEMP_SB"
  Data Type Conversion70/1 -> Bus Creator/65  "bsw_65_EV_MOT_PHASE_V_OFFSET"
  Data Type Conversion68/1 -> Bus Creator/63  "bsw_63_EV_MOT_PHASE_CHECK_ERROR"
  Data Type Conversion69/1 -> Bus Creator/64  "bsw_64_EV_MOT_PHASE_U_OFFSET"
  Data Type Conversion67/1 -> Bus Creator/62  "bsw_62_EV_MOT_PHASE_W_SW_OC"
  Data Type Conversion71/1 -> Bus Creator/66  "bsw_66_EV_MOT_PHASE_W_OFFSET"
  Data Type Conversion74/1 -> Bus Creator/75  "bsw_75_EV_SIC_W_TEMP_OOR"
  Data Type Conversion73/1 -> Bus Creator/68  "bsw_68_EV_SIC_U_TEMP_SB"
  Data Type Conversion72/1 -> Bus Creator/67  "bsw_67_EV_SIC_U_TEMP_SGOP"
  Data Type Conversion76/1 -> Bus Creator/77  "bsw_77_EV_MOT_GFLT_VH"
  Data Type Conversion77/1 -> Bus Creator/78  "bsw_78_EV_MOT_GFLT_WH"
  Data Type Conversion78/1 -> Bus Creator/79  "bsw_79_EV_MOT_GFLT_UL"
  Data Type Conversion75/1 -> Bus Creator/76  "bsw_76_EV_MOT_GFLT_UH"
  Data Type Conversion82/1 -> Bus Creator/91  "bsw_91_EV_HV2DC_VOLT_SB"
  Data Type Conversion81/1 -> Bus Creator/90  "bsw_90_EV_HV2DC_VOLT_SGOP"
  Data Type Conversion79/1 -> Bus Creator/80  "bsw_80_EV_MOT_GFLT_VL"
  Data Type Conversion80/1 -> Bus Creator/81  "bsw_81_EV_MOT_GFLT_WL"
  Data Type Conversion83/1 -> Bus Creator/92  "bsw_92_EV_HV2DC_VOLT_OOR"
  Data Type Conversion84/1 -> Bus Creator/93  "bsw_93_PCB_TEMP1_SGOP"
  Data Type Conversion85/1 -> Bus Creator/94  "bsw_94_PCB_TEMP1_SB"
  Data Type Conversion87/1 -> Bus Creator/82  "bsw_82_EV_MOT1_INVERTER_CRIT_OT"
  Data Type Conversion88/1 -> Bus Creator/83  "bsw_83_EV_MOT1_INVERTER_OT"
  Data Type Conversion86/1 -> Bus Creator/95  "bsw_95_PCB_TEMP2_SGOP"
  Data Type Conversion90/1 -> Bus Creator/85  "bsw_85_EV_HVDC_VOLT_LO"
  Data Type Conversion91/1 -> Bus Creator/86  "bsw_86_EV_HVDC_VOLT_HI"
  Data Type Conversion92/1 -> Bus Creator/87  "bsw_87_EV_HV1DC_VOLT_SGOP"
  Data Type Conversion95/1 -> Bus Creator/96  "bsw_96_PCB_TEMP2_SB"
  Data Type Conversion89/1 -> Bus Creator/84  "bsw_84_EV_HVDC_VOLT_HW_OV"
  Data Type Conversion93/1 -> Bus Creator/88  "bsw_88_EV_HV1DC_VOLT_SB"
  Data Type Conversion94/1 -> Bus Creator/89  "bsw_89_EV_HV1DC_VOLT_OOR"
  Data Type Conversion101/1 -> Bus Creator/108  "bsw_108_KL30_Backup_OOR"
  Data Type Conversion100/1 -> Bus Creator/107  "bsw_107_KL30_Backup_HI"
  Data Type Conversion99/1 -> Bus Creator/106  "bsw_106_KL30_Backup_LO"
  Data Type Conversion102/1 -> Bus Creator/97  "bsw_97_PCB_TEMP_OT"
  Data Type Conversion104/1 -> Bus Creator/99  "bsw_99_Oil_TEMP_SB"
  Data Type Conversion103/1 -> Bus Creator/98  "bsw_98_Oil_TEMP_SGOP"
  Data Type Conversion108/1 -> Bus Creator/109  "bsw_109_IGN_Vol_LO"
  Data Type Conversion107/1 -> Bus Creator/102  "bsw_102_KL30_UV"
  Data Type Conversion106/1 -> Bus Creator/101  "bsw_101_water_TEMP_OT"
  Data Type Conversion105/1 -> Bus Creator/100  "bsw_100_Oil_TEMP_OT"
  Data Type Conversion98/1 -> Bus Creator/105  "bsw_105_KL31_SB"
  Data Type Conversion96/1 -> Bus Creator/103  "bsw_103_KL30_OV"
  Data Type Conversion97/1 -> Bus Creator/104  "bsw_104_KL30_SGOP"
  Data Type Conversion112/1 -> Bus Creator/111  "bsw_111_VPREREG_OOR"
  Data Type Conversion111/1 -> Bus Creator/110  "bsw_110_IGN_Vol_HI"
  Data Type Conversion115/1 -> Bus Creator/114  "bsw_114_VCC5V_CAN_OOR"
  Data Type Conversion109/1 -> Bus Creator/120  "bsw_120_VCC5VUC_OOR"
  Data Type Conversion113/1 -> Bus Creator/112  "bsw_112_VPREREG_SGOP"
  Data Type Conversion110/1 -> Bus Creator/121  "bsw_121_VCC5VUC_SGOP"
  Data Type Conversion114/1 -> Bus Creator/113  "bsw_113_VPREREG_SB"
  Data Type Conversion117/1 -> Bus Creator/122  "bsw_122_VCC5VUC_SB"
  Data Type Conversion118/1 -> Bus Creator/116  "bsw_116_VCC5V_CAN_SB"
  Data Type Conversion116/1 -> Bus Creator/115  "bsw_115_VCC5V_CAN_SGOP"
  Data Type Conversion120/1 -> Bus Creator/118  "bsw_118_VREF5V_SGOP"
  Data Type Conversion119/1 -> Bus Creator/117  "bsw_117_VREF5V_OOR"
  Data Type Conversion121/1 -> Bus Creator/119  "bsw_119_VREF5V_SB"
  Data Type Conversion129/1 -> Bus Creator/128  "bsw_128_VCC5VT2_SB"
  Data Type Conversion127/1 -> Bus Creator/126  "bsw_126_VCC5VT2_5V_OOR"
  Data Type Conversion132/1 -> Bus Creator/130  "bsw_130_VCC5V_GDL_OOR"
  Data Type Conversion131/1 -> Bus Creator/129  "bsw_129_VCC5V_GDH_OOR"
  Data Type Conversion124/1 -> Bus Creator/123  "bsw_123_VCC5VT1_OOR"
  Data Type Conversion125/1 -> Bus Creator/124  "bsw_124_VCC5VT1_SGOP"
  Data Type Conversion128/1 -> Bus Creator/127  "bsw_127_VCC5VT2_SGOP"
  Data Type Conversion126/1 -> Bus Creator/125  "bsw_125_VCC5VT1_SB"
  Demux/132 -> Mux/1
  Demux/133 -> Mux/2
  Demux/134 -> Mux/3
  Demux/135 -> Mux/4
  Demux/136 -> Mux/5
  Demux/137 -> Mux/6
  Demux/138 -> Mux/7
  Demux/139 -> Mux/8
  Demux/140 -> Mux/9
  Demux/141 -> Mux/10
  Demux/142 -> Mux/11
  Demux/143 -> Mux/12
  Demux/144 -> Mux/13
  Demux/145 -> Mux/14
  Demux/146 -> Mux/15
  Demux/147 -> Mux/16
  Demux/148 -> Mux/17
  Demux/149 -> Mux/18
  Demux/150 -> Mux/19
  Mux/1 -> Terminator1/1

== system dgl_grc/Subsystem/EOPSpeedMonitor ==
  note: EOP转速监控
  EOPC_nEOPSpdAct : Inport  OutDataTypeStr=single
  EOPC_nEOPSpdReq : Inport  Port=2  OutDataTypeStr=single
  Abs : Abs  SaturateOnIntegerOverflow=off
  Constant1 : Constant  Value=KDGL_tiDlyOnEOP_C
  Constant18 : Constant  Value=GRC_FAKE_SAMPLE_TIME
  Constant20 : Constant  Value=KDGL_tiDlyOffEOP_C
  Constant35 : Constant  Value=KDGL_nEOPSpdDiff_rpm
  Constant38 : Constant  Value=GRC_FAKE_SAMPLE_TIME
  Relational Operator1 : RelationalOperator  OutDataTypeStr=boolean  RndMeth=Simplest  InputSameDT=off
  Subtract : Sum  Inputs=+-
  TurnOffDelay_Dyn1 : GRC_Lib/Delay/TurnOffDelay_Dyn  IpDT=single
  TurnOnDelay_Dyn2 : GRC_Lib/Delay/TurnOnDelay_Dyn  IpDT=single
  DiagM_bEOPFlt : Outport  VectorParamsAs1DForOutWhenUnconnected=off
  wires:
  Relational Operator1/1 -> TurnOnDelay_Dyn2/1
  Constant20/1 -> TurnOffDelay_Dyn1/2
  TurnOffDelay_Dyn1/1 -> DiagM_bEOPFlt/1  "DiagM_bEOPFlt"
  Constant18/1 -> TurnOffDelay_Dyn1/3
  Constant35/1 -> Relational Operator1/2
  Constant38/1 -> TurnOnDelay_Dyn2/3
  TurnOnDelay_Dyn2/1 -> TurnOffDelay_Dyn1/1
  EOPC_nEOPSpdReq/1 -> Subtract/1
  Constant1/1 -> TurnOnDelay_Dyn2/2
  EOPC_nEOPSpdAct/1 -> Subtract/2
  Subtract/1 -> Abs/1
  Abs/1 -> Relational Operator1/1

== system dgl_grc/Subsystem/OverLowVolDerate ==
  DSS_uDCSide : Inport  OutDataTypeStr=single
  ModControl : Inport  Port=2  OutDataTypeStr=uint8
  BMS_bContactorClsd : Inport  Port=3  OutDataTypeStr=boolean
  Bus Creator : BusCreator  Inputs=2
  HVLowMonitor : Subsystem
  HVOverMonitor : Subsystem
  HV_Out : Outport  VectorParamsAs1DForOutWhenUnconnected=off
  wires:
  DSS_uDCSide/1 -> HVLowMonitor/1(Udc), HVOverMonitor/1(Udc)
  ModControl/1 -> HVLowMonitor/2(ModControl)
  BMS_bContactorClsd/1 -> HVLowMonitor/3(BMS_bContactorClsd)
  HVOverMonitor/1(Out) -> Bus Creator/1  "HVOverMonitor"
  HVLowMonitor/1(Out) -> Bus Creator/2  "HVLowMonitor"
  Bus Creator/1 -> HV_Out/1

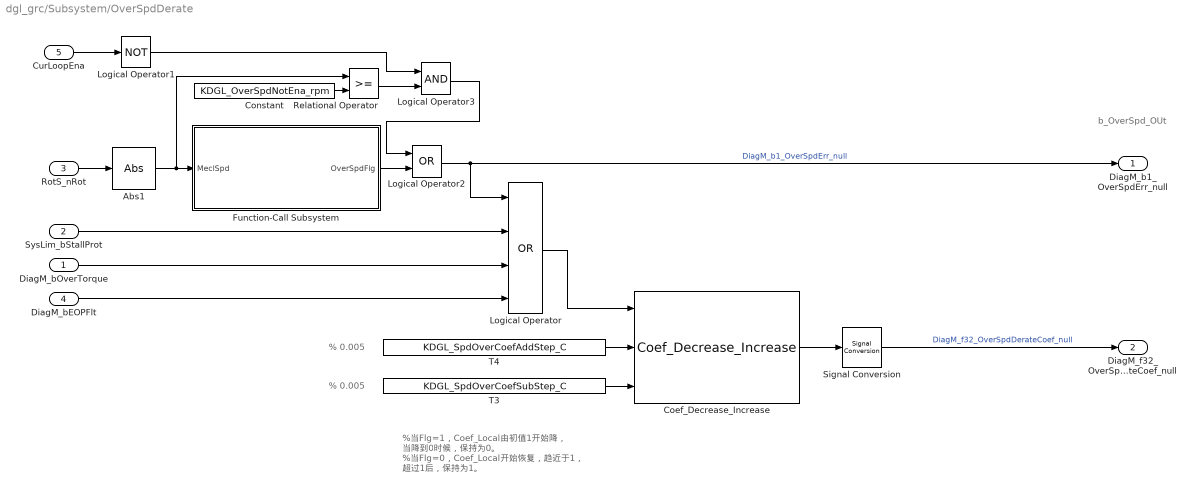
== system dgl_grc/Subsystem/OverSpdDerate ==
  note: b_OverSpd_OUt
  note: % 0.005
  note: % 0.005
  note: %当Flg=1，Coef_Local由初值1开始降，
      | 当降到0时候，保持为0。
      | %当Flg=0，Coef_Local开始恢复，趋近于1，
      | 超过1后，保持为1。
  DiagM_bOverTorque : Inport
  SysLim_bStallProt : Inport  Port=2
  RotS_nRot : Inport  Port=3  OutDataTypeStr=single
  DiagM_bEOPFlt : Inport  Port=4  OutDataTypeStr=boolean
  CurLoopEna : Inport  Port=5
  Abs1 : Library/Abs  SystemSampleTime=-1  VariantActivationTime=update diagram  AllowFlexibleInterface=on  Latency=0  AutoFrameSizeCalculation=off
  Coef_Decrease_Increase : Library/Coef_Decrease_Increase  SystemSampleTime=-1  VariantActivationTime=update diagram  AllowFlexibleInterface=on  Latency=0  AutoFrameSizeCalculation=off
  Constant : Constant  Value=KDGL_OverSpdNotEna_rpm  OutDataTypeStr=single
  Function-Call Subsystem : Subsystem  TreatAsAtomicUnit=on
  Logical Operator : Logic  Operator=OR  Inputs=4  AllPortsSameDT=off  OutDataTypeStr=boolean
  Logical Operator1 : Logic  Operator=NOT  AllPortsSameDT=off  OutDataTypeStr=boolean
  Logical Operator2 : Logic  Operator=OR  AllPortsSameDT=off  OutDataTypeStr=boolean
  Logical Operator3 : Logic  AllPortsSameDT=off  OutDataTypeStr=boolean
  Relational Operator : RelationalOperator  OutDataTypeStr=boolean  RndMeth=Simplest  InputSameDT=off
  Signal Conversion : SignalConversion  OverrideOpt=off
  T3 : Constant  Value=KDGL_SpdOverCoefSubStep_C  OutDataTypeStr=single
  T4 : Constant  Value=KDGL_SpdOverCoefAddStep_C  OutDataTypeStr=single
  DiagM_b1_OverSpdErr_null : Outport  VectorParamsAs1DForOutWhenUnconnected=off
  DiagM_f32_OverSpdDerateCoef_null : Outport  Port=2  VectorParamsAs1DForOutWhenUnconnected=off
  wires:
  Coef_Decrease_Increase/1 -> Signal Conversion/1
  Signal Conversion/1 -> DiagM_f32_OverSpdDerateCoef_null/1  "DiagM_f32_OverSpdDerateCoef_null"
  Abs1/1 -> Relational Operator/1, Function-Call Subsystem/1(MeclSpd)
  Logical Operator2/1 -> Logical Operator/1, DiagM_b1_OverSpdErr_null/1  "DiagM_b1_OverSpdErr_null"
  T3/1 -> Coef_Decrease_Increase/3
  T4/1 -> Coef_Decrease_Increase/2
  RotS_nRot/1 -> Abs1/1
  SysLim_bStallProt/1 -> Logical Operator/2
  Logical Operator/1 -> Coef_Decrease_Increase/1
  DiagM_bOverTorque/1 -> Logical Operator/3
  DiagM_bEOPFlt/1 -> Logical Operator/4
  CurLoopEna/1 -> Logical Operator1/1
  Logical Operator1/1 -> Logical Operator3/1
  Logical Operator3/1 -> Logical Operator2/1
  Function-Call Subsystem/1(OverSpdFlg) -> Logical Operator2/2
  Constant/1 -> Relational Operator/2
  Relational Operator/1 -> Logical Operator3/2
